simulink model "LC_control"  (R2023b)
settings: configuration reference "slow_tsk_conf" (kept outside this file)
settings Model: DataDictionary=fmuGenerationDictionay.sldd  Creator=Veimar  LastModifiedBy=Veimar
settings ConfigSetRef: SourceName=slow_tsk_conf

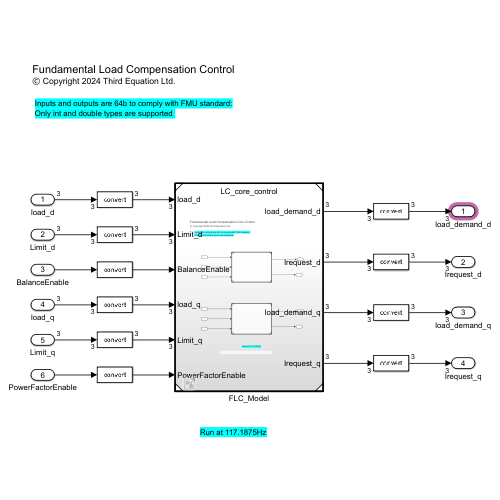
[thumbnail: Simulink's stored preview of the top-level diagram]
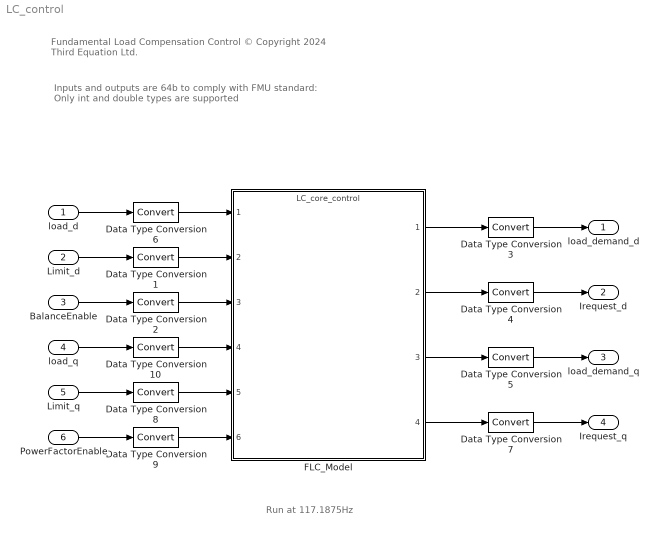
== system LC_control ==
  note: Fundamental Load Compensation Control
      | © Copyright 2024 Third Equation Ltd.
  note: Inputs and outputs are 64b to comply with FMU standard:
      | Only int and double types are supported
  note: Run at 117.1875Hz
  load_d : Inport  OutDataTypeStr=double  PortDimensions=3
  Limit_d : Inport  Port=2  OutDataTypeStr=double  PortDimensions=3
  BalanceEnable : Inport  Port=3  OutDataTypeStr=int64  PortDimensions=1
  load_q : Inport  Port=4  OutDataTypeStr=double  PortDimensions=3
  Limit_q : Inport  Port=5  OutDataTypeStr=double  PortDimensions=3
  PowerFactorEnable : Inport  Port=6  OutDataTypeStr=int64  PortDimensions=1
  Data Type Conversion{1..10} (10 alike) : DataTypeConversion  SaturateOnIntegerOverflow=off  RndMeth=Floor
  FLC_Model : ModelReference  ModelNameDialog=LC_core_control.slx  SimulationMode=Normal  ModelReferenceVersion=1.18
  load_demand_d : Outport  OutDataTypeStr=double  PortDimensions=3
  Irequest_d : Outport  Port=2  OutDataTypeStr=double  PortDimensions=3
  load_demand_q : Outport  Port=3  OutDataTypeStr=double  PortDimensions=3
  Irequest_q : Outport  Port=4  OutDataTypeStr=double  PortDimensions=3
  wires:
  load_d/1 -> Data Type Conversion6/1
  Data Type Conversion6/1 -> FLC_Model/1
  Limit_d/1 -> Data Type Conversion1/1
  Data Type Conversion1/1 -> FLC_Model/2
  BalanceEnable/1 -> Data Type Conversion2/1
  Data Type Conversion2/1 -> FLC_Model/3
  FLC_Model/1 -> Data Type Conversion3/1
  FLC_Model/2 -> Data Type Conversion4/1
  Data Type Conversion3/1 -> load_demand_d/1
  Data Type Conversion4/1 -> Irequest_d/1
  Data Type Conversion7/1 -> Irequest_q/1
  Data Type Conversion5/1 -> load_demand_q/1
  FLC_Model/4 -> Data Type Conversion7/1
  FLC_Model/3 -> Data Type Conversion5/1
  Limit_q/1 -> Data Type Conversion8/1
  Data Type Conversion8/1 -> FLC_Model/5
  Data Type Conversion10/1 -> FLC_Model/4
  Data Type Conversion9/1 -> FLC_Model/6
  PowerFactorEnable/1 -> Data Type Conversion9/1
  load_q/1 -> Data Type Conversion10/1
